simulink model "segbpp"  (R2020b)
settings: Solver=VariableStepAuto  StartTime=0.0  StopTime=100  RelTol=1e-3
settings Model: Creator=Acer  LastModifiedBy=Acer

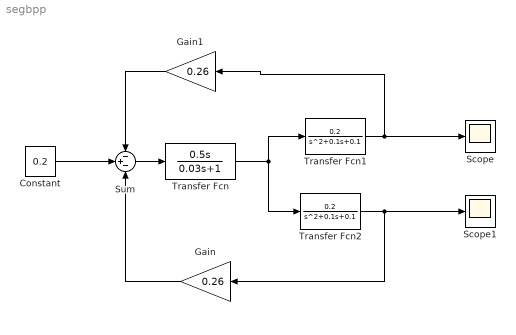
== system segbpp ==
  Constant : Constant  Value=0.2
  Gain : Gain  Gain=0.26
  Gain1 : Gain  Gain=0.26
  Scope : Scope
  Scope1 : Scope
  Sum : Sum  Inputs=-+-
  Transfer Fcn : TransferFcn  Numerator=[0.5 0]  Denominator=[0.03 1]
  Transfer Fcn1 : TransferFcn  Numerator=[0.2]  Denominator=[1 0.1 0.1]
  Transfer Fcn2 : TransferFcn  Numerator=[0.2]  Denominator=[1 0.1 0.1]
  wires:
  Gain/1 -> Sum/3
  Gain1/1 -> Sum/1
  Sum/1 -> Transfer Fcn/1
  Transfer Fcn/1 -> Transfer Fcn2/1, Transfer Fcn1/1
  Transfer Fcn1/1 -> Scope/1, Gain1/1
  Transfer Fcn2/1 -> Scope1/1, Gain/1
  Constant/1 -> Sum/2
